simulink model "sampleModel141"  (R2021b)
settings: Solver=VariableStepAuto  StartTime=0.0  StopTime=10.0  RelTol=1e-3
undefined symbols (not defined in the file or in its folder): DiscIntNeverNeededParam
libraries: simulink x4, slpidlib x1
settings Model: Creator=user  LastModifiedBy=user

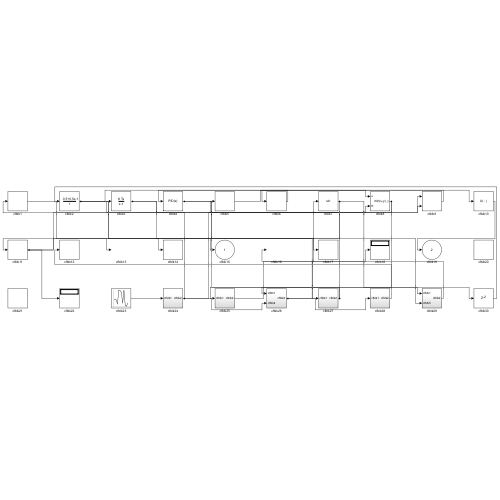
[thumbnail: Simulink's stored preview of the top-level diagram]
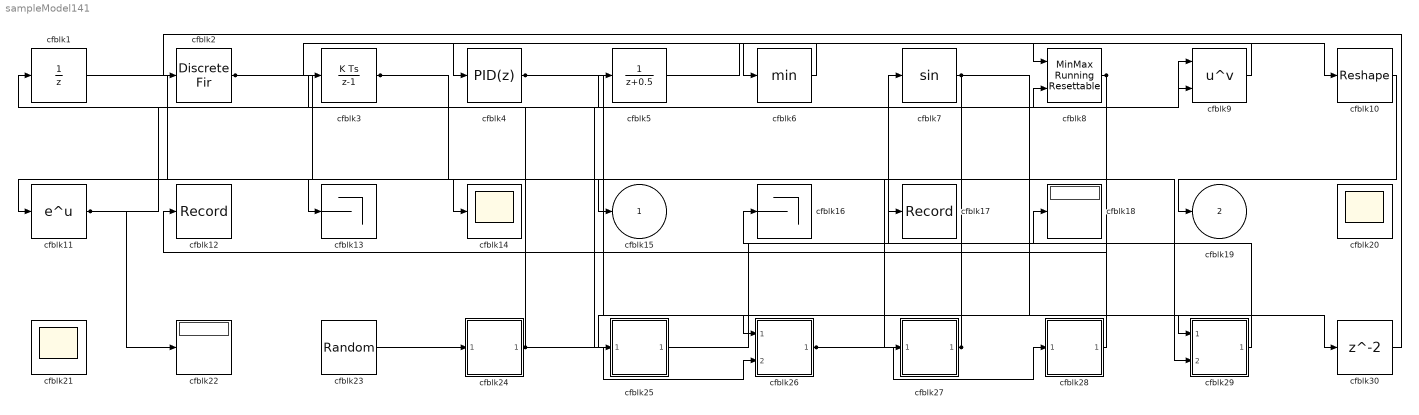
== system sampleModel141 ==
  cfblk1 : UnitDelay  HasFrameUpgradeWarning=on
  cfblk10 : Reshape
  cfblk11 : Math  SaturateOnIntegerOverflow=on
  cfblk12 : Record  FileSettingsInternal="{\"entries\":[{\"content\":{\"excelSettings\":{\"content\":{},\"type\":\"Streamout.ExcelSettings\"}},\"type\":\"Streamout.FileSettingStorage\",\"uuid\":\"a39cff4f-daf2-4c28-a5b7-ec255e5ac0f6\"}],\"packageUris\":[\"http://schema.mathworks.com/mf0/streamout_blocks/R2020a\"],\"version\":\"1.0\"}"  SignalsInternal="{\"entries\":[{\"content\":{\"signals\":[{\"content\":{\"blockPath\":[\"sampleModel141/cfblk12\"],\"channel\":[],\"dimensions\":[1],\"domain\":\"sampleModel141/cfblk12\",\"lineColor\":\"#77ac30\",\"plots\":[1],\"port\":1,\"sid\":[\"\"],\"signalID\":5043,\"signalName\":\"cfblk28\"},\"type\":\"RecordBlkView.Signal\",\"uuid\":\"52644dd1-6354-4493-8342-73fe0015a786\"}]},\"type\":\"RecordBlkView.InputSignals\",\"uuid\":\"56e0f7c8-4d96-4cb7-bdb7-98e7153dadd1\"}],\"packageUris\":[\"http://schema.mathworks.com/mf0/streamout_blocks/R2020a\"],\"version\":\"1.0\"}"  VisualizationBindings="{\"sparklinesplugin\":{\"info\":[{\"bindingParametersList\":[],\"subplotID\":1}]}}"
  cfblk13 : Terminator
  cfblk14 : Scope
  cfblk16 : Terminator
  cfblk17 : Record  FileSettingsInternal="{\"entries\":[{\"content\":{\"excelSettings\":{\"content\":{},\"type\":\"Streamout.ExcelSettings\"}},\"type\":\"Streamout.FileSettingStorage\",\"uuid\":\"e404dd9b-bba9-46a7-9a10-97498adcddd8\"}],\"packageUris\":[\"http://schema.mathworks.com/mf0/streamout_blocks/R2020a\"],\"version\":\"1.0\"}"  SignalsInternal="{\"entries\":[{\"content\":{\"signals\":[{\"content\":{\"blockPath\":[\"sampleModel141/cfblk17\"],\"channel\":[],\"dimensions\":[1],\"domain\":\"sampleModel141/cfblk17\",\"lineColor\":\"#4dbeee\",\"plots\":[1],\"port\":1,\"sid\":[\"\"],\"signalID\":5047,\"signalName\":\"cfblk3\"},\"type\":\"RecordBlkView.Signal\",\"uuid\":\"1d29c7ec-9dd9-4208-8596-fda88c1fd611\"}]},\"type\":\"RecordBlkView.InputSignals\",\"uuid\":\"7f42791e-e920-4f00-9e91-acc0e9c6bbc6\"}],\"packageUris\":[\"http://schema.mathworks.com/mf0/streamout_blocks/R2020a\"],\"version\":\"1.0\"}"  VisualizationBindings="{\"sparklinesplugin\":{\"info\":[{\"bindingParametersList\":[],\"subplotID\":1}]}}"
  cfblk18 : Display
  cfblk2 : DiscreteFir  SampleTime=1
  cfblk20 : Scope
      settings: Floating=on
  cfblk21 : Scope
      settings: Floating=on
  cfblk22 : Display
  cfblk23 : RandomNumber  Mean=[51555.156439]  Variance=[47411.369966]  Seed=[690428430.000000]  SampleTime=0.1
  cfblk24 : Subsystem
  cfblk25 : Subsystem
  cfblk26 : Subsystem
  cfblk27 : Subsystem
  cfblk28 : Subsystem
  cfblk29 : Subsystem
  cfblk3 : DiscreteIntegrator  ICPrevOutput=DiscIntNeverNeededParam  ICPrevScaledInput=DiscIntNeverNeededParam
  cfblk30 : Delay  SampleTime=1
  cfblk4 : slpidlib/PID Controller  Controller=PID  Form=Parallel  TimeDomain=Discrete-time  UseExternalTs=off  SampleTime=1  IntegratorMethod=Forward Euler  FilterMethod=Forward Euler  ControllerParametersSource=internal  P=1  I=1  D=0  UseFilter=on  N=100  TunerSelectOption=Transfer Function Based (PID Tuner App)  InitialConditionSource=internal  InitialConditionForIntegrator=0  InitialConditionForFilter=0  DifferentiatorICPrevScaledInput=0  ExternalReset=none  TrackingMode=off  Kt=1  LimitOutput=off  SatLimitsSource=internal  UpperSaturationLimit=inf  LowerSaturationLimit=-inf  LinearizeAsGain=off  AntiWindupMode=none  Kb=1  POutMin=[]  POutMax=[]  IOutMin=[]  IOutMax=[]  DOutMin=[]  DOutMax=[]  NOutMin=[]  NOutMax=[]  SumOutMin=[]  SumOutMax=[]  SaturationOutMin=[]  SaturationOutMax=[]  PParamMin=[]  PParamMax=[]  IParamMin=[]  IParamMax=[]  DParamMin=[]  DParamMax=[]  NParamMin=[]  NParamMax=[]  KbParamMin=[]  KbParamMax=[]  KtParamMin=[]  KtParamMax=[]  KbOutMin=[]  KbOutMax=[]  KtOutMin=[]  KtOutMax=[]  IntegratorOutMin=[]  IntegratorOutMax=[]  FilterOutMin=[]  FilterOutMax=[]  SumI1OutMin=[]  SumI1OutMax=[]  SumI2OutMin=[]  SumI2OutMax=[]  SumI3OutMin=[]  SumI3OutMax=[]  SumI4OutMin=[]  SumI4OutMax=[]  SumDOutMin=[]  SumDOutMax=[]  DifferentiatorOutMin=[]  DifferentiatorOutMax=[]  FilterDiffOutCoefMin=[]  FilterDiffOutCoefMax=[]  ReciprocalOutMin=[]  ReciprocalOutMax=[]  SumDenOutMin=[]  SumDenOutMax=[]  SumNumOutMin=[]  SumNumOutMax=[]  DivideOutMin=[]  DivideOutMax=[]  UdiffTsProdOutMin=[]  UdiffTsProdOutMax=[]  NTsProdOutMin=[]  NTsProdOutMax=[]  UintegralTsProdOutMin=[]  UintegralTsProdOutMax=[]  UngainTsProdOutMin=[]  UngainTsProdOutMax=[]  IntegratorContinuousStateAttributes=''  IntegratorStateMustResolveToSignalObject=off  IntegratorRTWStateStorageClass=Auto  FilterContinuousStateAttributes=''  FilterStateMustResolveToSignalObject=off  FilterRTWStateStorageClass=Auto  ParallelPVariant=InternalParameters  IdealPVariant=Disabled  IVariant=InternalParameters  DVariant=InternalParameters  IntegratorVariant=Discrete  SatVariant=Disabled  AWVariant=Passthrough  PCopyVariant=Disabled  TRVariant=Disabled  FdbkBlocksVariant=Forward  IdealPFdbkVariant=Disabled  SatFdbkVariant=Disabled  DerivativeFilterVariant=ForwardEulerFilter  NVariant=InternalParameters  NCopyVariant=Disabled  FilterICVariant=InternalICsFilter  IntegratorICVariant=InternalICs  ExternalResetVariant=Disabled  TRSumVariant=Passthrough  SumFdbkVariant=Disabled  SumVariant=Sum_PID  TsampFilterVariant=InternalTs  TsampNgainVariant=Passthrough  TsampIntegralVariant=Passthrough  ExternalSaturationOutDataTypeStr=Inherit: Same as second input
  cfblk5 : DiscreteTransferFcn  SampleTime=1
  cfblk6 : MinMax
  cfblk7 : Trigonometry
  cfblk8 : simulink/Math Operations/MinMax Running Resettable  Function=min  vinit=0.0
  cfblk9 : Math  Operator=pow  SaturateOnIntegerOverflow=on
  cfblk15 : Outport
  cfblk19 : Outport  Port=2
  wires:
  cfblk6/1 -> cfblk4/1
  cfblk29/1(cfblk2) -> cfblk16/1
  cfblk10/1 -> cfblk19/1
  cfblk11/1 -> cfblk22/1, cfblk9/1, cfblk14/1
  cfblk8/1 -> cfblk1/1, cfblk25/1(cfblk1)
  cfblk1/1 -> cfblk13/1
  cfblk28/1(cfblk2) -> cfblk12/1
  cfblk25/1(cfblk2) -> cfblk7/1
  cfblk3/1 -> cfblk17/1, cfblk8/2
  cfblk23/1 -> cfblk24/1(cfblk1)
  cfblk9/1 -> cfblk6/1
  cfblk4/1 -> cfblk29/1(cfblk1), cfblk29/2(cfblk5)
  cfblk27/1(cfblk2) -> cfblk26/1(cfblk1), cfblk5/1
  cfblk7/1 -> cfblk11/1, cfblk30/1
  cfblk24/1(cfblk2) -> cfblk26/2(cfblk4), cfblk9/2, cfblk3/1
  cfblk5/1 -> cfblk8/1
  cfblk2/1 -> cfblk15/1, cfblk27/1(cfblk1), cfblk10/1
  cfblk26/1(cfblk2) -> cfblk28/1(cfblk1), cfblk18/1
  cfblk30/1 -> cfblk2/1

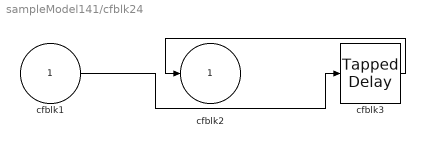
== system sampleModel141/cfblk24 ==
  cfblk1 : Inport
  cfblk3 : simulink/Discrete/Tapped Delay  vinit=0.0  samptime=-1  NumDelays=1  DelayOrder=Oldest  includeCurrent=off
  cfblk2 : Outport
  wires:
  cfblk3/1 -> cfblk2/1
  cfblk1/1 -> cfblk3/1

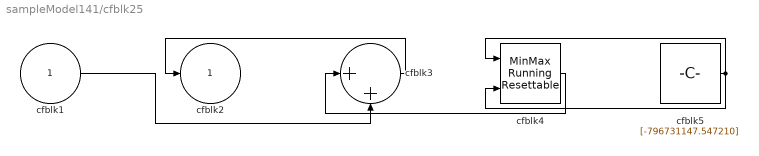
== system sampleModel141/cfblk25 ==
  cfblk1 : Inport
  cfblk3 : Sum  Inputs=|++
  cfblk4 : simulink/Math Operations/MinMax Running Resettable  Function=min  vinit=0.0
  cfblk5 : Constant  Value=[-796731147.547210]  SampleTime=1
  cfblk2 : Outport
  wires:
  cfblk3/1 -> cfblk2/1
  cfblk5/1 -> cfblk4/1, cfblk4/2
  cfblk4/1 -> cfblk3/1
  cfblk1/1 -> cfblk3/2

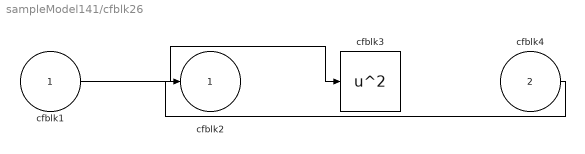
== system sampleModel141/cfblk26 ==
  cfblk1 : Inport
  cfblk4 : Inport  Port=2
  cfblk3 : Math  Operator=square  SaturateOnIntegerOverflow=on
  cfblk2 : Outport
  wires:
  cfblk1/1 -> cfblk3/1
  cfblk4/1 -> cfblk2/1

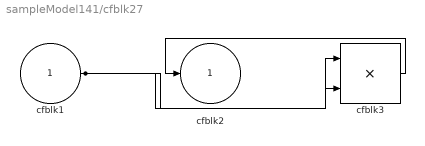
== system sampleModel141/cfblk27 ==
  cfblk1 : Inport
  cfblk3 : Product  Inputs=**
  cfblk2 : Outport
  wires:
  cfblk3/1 -> cfblk2/1
  cfblk1/1 -> cfblk3/1, cfblk3/2

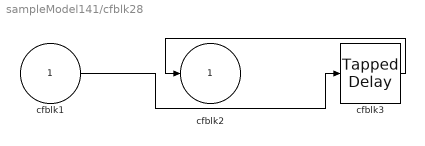
== system sampleModel141/cfblk28 ==
  cfblk1 : Inport
  cfblk3 : simulink/Discrete/Tapped Delay  vinit=0.0  samptime=-1  NumDelays=1  DelayOrder=Oldest  includeCurrent=off
  cfblk2 : Outport
  wires:
  cfblk3/1 -> cfblk2/1
  cfblk1/1 -> cfblk3/1

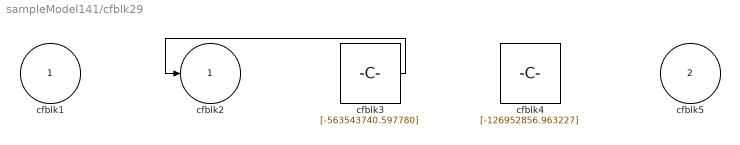
== system sampleModel141/cfblk29 ==
  cfblk1 : Inport
  cfblk5 : Inport  Port=2
  cfblk3 : Constant  Value=[-563543740.597780]  SampleTime=1
  cfblk4 : Constant  Value=[-126952856.963227]  SampleTime=1
  cfblk2 : Outport
  wires:
  cfblk3/1 -> cfblk2/1
